simulink model "S205_Anwendungsbeispiel"  (R2018b)
settings: Solver=VariableStepAuto  StartTime=0.0  StopTime=10  MaxStep=0.001  RelTol=1e-3
values from neighbouring files (symbols this model uses):
  a = 0.031    [Parameter_S205.m]
  c = 1160    [Parameter_S205.m]
  d = 0.6    [Parameter_S205.m]
  delta_ksi = (20-(-20))/(2*r-1)    (= 1.37931034483)    [Parameter_S205.m]
  eta_c = 5*10^4    (= 50000)    [Parameter_S205.m]
  eta_d = 1.25    [Parameter_S205.m]
  eta_J1 = 0.15    [Parameter_S205.m]
  eta_J2 = 4*10^(-3)    (= 0.004)    [Parameter_S205.m]
  eta_Reib1 = 0.125    [Parameter_S205.m]
  eta_Reib2 = 0.1    [Parameter_S205.m]
  eta_theta_L = 8*10^(-6)    (= 8e-06)    [Parameter_S205.m]
  h = 0.4*10^(-3)    (= 0.0004)    [Parameter_S205.m]
  J1 = 0.166    [Parameter_S205.m]
  J2 = 0.336    [Parameter_S205.m]
  ksi = linspace(-20,20,2*r)    [Parameter_S205.m]
  l1 = 3.3    [Parameter_S205.m]
  l2 = 2.6    [Parameter_S205.m]
  l4 = 98    [Parameter_S205.m]
  sigma_norm = 1.6    [Parameter_S205.m]
  theta_S1 = 2    [Parameter_S205.m]
  theta_S2 = 38    [Parameter_S205.m]
undefined symbols (not defined in the file or in its folder): DiscIntNeverNeededParam
libraries: simulink x1
settings Model: Creator=LENOVO  LastModifiedBy=LENOVO

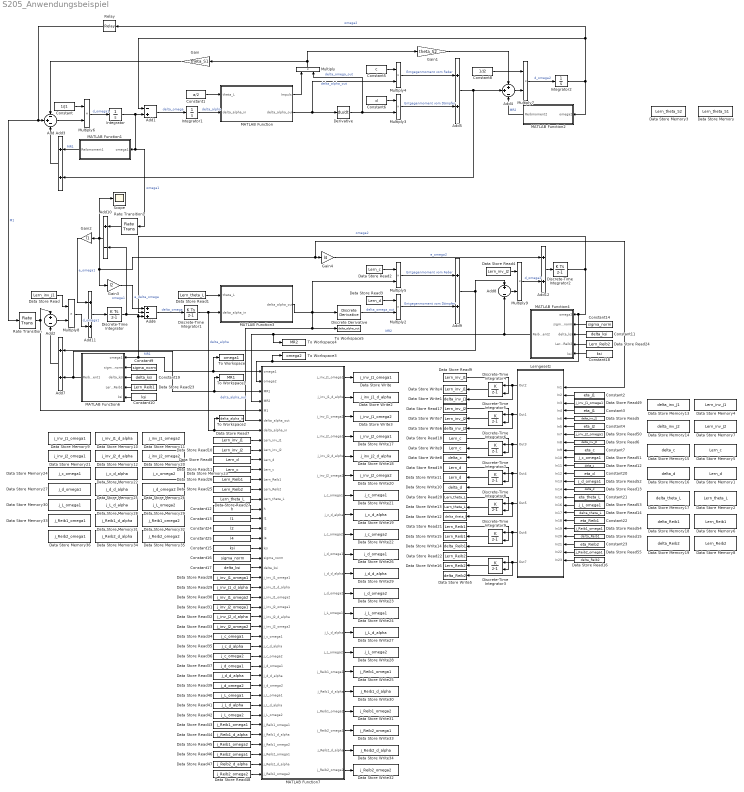
== system S205_Anwendungsbeispiel ==
  Add : Sum  Inputs=-+-
  Add1 : Sum  Inputs=-+
  Add10 : Sum  Inputs=+-
  Add{3,5,7,9,11..12} (6 alike) : Sum
  Add2 : Sum  Inputs=+-
  Add4 : Sum  Inputs=++-
  Add6 : Sum  Inputs=+-+
  Add8 : Sum  Inputs=+-
  Constant : Constant  Value=1/J1
  Constant1 : Constant  Value=a/2
  Constant10 : Constant  Value=ksi
  Constant11 : Constant  Value=delta_ksi
  Constant12 : Constant  Value=h
  Constant13 : Constant  Value=l1
  Constant14 : Constant  Value=sigma_norm
  Constant15 : Constant  Value=ksi
  Constant16 : Constant  Value=sigma_norm
  Constant17 : Constant  Value=delta_ksi
  Constant18 : Constant  Value=ksi
  Constant19 : Constant  Value=delta_ksi
  Constant2 : Constant  Value=eta_J1
  Constant20 : Constant  Value=eta_d
  Constant21 : Constant  Value=eta_theta_L
  Constant22 : Constant  Value=eta_Reib1
  Constant23 : Constant  Value=eta_Reib2
  Constant24 : Constant  Value=l2
  Constant25 : Constant  Value=l4
  Constant3 : Constant  Value=eta_J1
  Constant4 : Constant  Value=eta_J2
  Constant5 : Constant  Value=c
  Constant6 : Constant  Value=d
  Constant7 : Constant  Value=eta_c
  Constant8 : Constant  Value=1/J2
  Constant9 : Constant  Value=sigma_norm
  Data Store Memory : DataStoreMemory  DataStoreName=Lern_theta_S1  ReadBeforeWriteMsg=warning  WriteAfterWriteMsg=warning  WriteAfterReadMsg=warning  ShowAdditionalParam=off
  Data Store Memory1 : DataStoreMemory  DataStoreName=Lern_d  ReadBeforeWriteMsg=warning  WriteAfterWriteMsg=warning  WriteAfterReadMsg=warning  InitialValue=1  ShowAdditionalParam=off
  Data Store Memory10 : DataStoreMemory  DataStoreName=j_inv_J1_d_alpha  ReadBeforeWriteMsg=warning  WriteAfterWriteMsg=warning  WriteAfterReadMsg=warning  ShowAdditionalParam=off
  Data Store Memory11 : DataStoreMemory  DataStoreName=j_inv_J1_omega2  ReadBeforeWriteMsg=warning  WriteAfterWriteMsg=warning  WriteAfterReadMsg=warning  ShowAdditionalParam=off
  Data Store Memory12 : DataStoreMemory  DataStoreName=j_inv_J2_d_alpha  ReadBeforeWriteMsg=warning  WriteAfterWriteMsg=warning  WriteAfterReadMsg=warning  ShowAdditionalParam=off
  Data Store Memory13 : DataStoreMemory  DataStoreName=delta_inv_J1  ReadBeforeWriteMsg=warning  WriteAfterWriteMsg=warning  WriteAfterReadMsg=warning  ShowAdditionalParam=off
  Data Store Memory14 : DataStoreMemory  DataStoreName=delta_inv_J2  ReadBeforeWriteMsg=warning  WriteAfterWriteMsg=warning  WriteAfterReadMsg=warning  ShowAdditionalParam=off
  Data Store Memory15 : DataStoreMemory  DataStoreName=delta_c  ReadBeforeWriteMsg=warning  WriteAfterWriteMsg=warning  WriteAfterReadMsg=warning  ShowAdditionalParam=off
  Data Store Memory16 : DataStoreMemory  DataStoreName=delta_d  ReadBeforeWriteMsg=warning  WriteAfterWriteMsg=warning  WriteAfterReadMsg=warning  ShowAdditionalParam=off
  Data Store Memory17 : DataStoreMemory  DataStoreName=delta_theta_L  ReadBeforeWriteMsg=warning  WriteAfterWriteMsg=warning  WriteAfterReadMsg=warning  ShowAdditionalParam=off
  Data Store Memory18 : DataStoreMemory  DataStoreName=delta_Reib1  ReadBeforeWriteMsg=warning  WriteAfterWriteMsg=warning  WriteAfterReadMsg=warning  InitialValue=zeros(1,30)  ShowAdditionalParam=off
  Data Store Memory19 : DataStoreMemory  DataStoreName=delta_Reib2  ReadBeforeWriteMsg=warning  WriteAfterWriteMsg=warning  WriteAfterReadMsg=warning  InitialValue=zeros(1,30)  ShowAdditionalParam=off
  Data Store Memory2 : DataStoreMemory  DataStoreName=Lern_theta_L  ReadBeforeWriteMsg=warning  WriteAfterWriteMsg=warning  WriteAfterReadMsg=warning  ShowAdditionalParam=off
  Data Store Memory20 : DataStoreMemory  DataStoreName=j_inv_J2_omega2  ReadBeforeWriteMsg=warning  WriteAfterWriteMsg=warning  WriteAfterReadMsg=warning  ShowAdditionalParam=off
  Data Store Memory21 : DataStoreMemory  DataStoreName=j_inv_J2_omega1  ReadBeforeWriteMsg=warning  WriteAfterWriteMsg=warning  WriteAfterReadMsg=warning  ShowAdditionalParam=off
  Data Store Memory22 : DataStoreMemory  DataStoreName=j_c_d_alpha  ReadBeforeWriteMsg=warning  WriteAfterWriteMsg=warning  WriteAfterReadMsg=warning  ShowAdditionalParam=off
  Data Store Memory23 : DataStoreMemory  DataStoreName=j_c_omega2  ReadBeforeWriteMsg=warning  WriteAfterWriteMsg=warning  WriteAfterReadMsg=warning  ShowAdditionalParam=off
  Data Store Memory24 : DataStoreMemory  DataStoreName=j_c_omega1  ReadBeforeWriteMsg=warning  WriteAfterWriteMsg=warning  WriteAfterReadMsg=warning  ShowAdditionalParam=off
  Data Store Memory25 : DataStoreMemory  DataStoreName=j_d_d_alpha  ReadBeforeWriteMsg=warning  WriteAfterWriteMsg=warning  WriteAfterReadMsg=warning  ShowAdditionalParam=off
  Data Store Memory26 : DataStoreMemory  DataStoreName=j_d_omega2  ReadBeforeWriteMsg=warning  WriteAfterWriteMsg=warning  WriteAfterReadMsg=warning  ShowAdditionalParam=off
  Data Store Memory27 : DataStoreMemory  DataStoreName=j_d_omega1  ReadBeforeWriteMsg=warning  WriteAfterWriteMsg=warning  WriteAfterReadMsg=warning  ShowAdditionalParam=off
  Data Store Memory28 : DataStoreMemory  DataStoreName=j_L_d_alpha  ReadBeforeWriteMsg=warning  WriteAfterWriteMsg=warning  WriteAfterReadMsg=warning  ShowAdditionalParam=off
  Data Store Memory29 : DataStoreMemory  DataStoreName=j_L_omega2  ReadBeforeWriteMsg=warning  WriteAfterWriteMsg=warning  WriteAfterReadMsg=warning  ShowAdditionalParam=off
  Data Store Memory3 : DataStoreMemory  DataStoreName=Lern_theta_S2  ReadBeforeWriteMsg=warning  WriteAfterWriteMsg=warning  WriteAfterReadMsg=warning  ShowAdditionalParam=off
  Data Store Memory30 : DataStoreMemory  DataStoreName=j_L_omega1  ReadBeforeWriteMsg=warning  WriteAfterWriteMsg=warning  WriteAfterReadMsg=warning  ShowAdditionalParam=off
  Data Store Memory31 : DataStoreMemory  DataStoreName=j_Reib1_d_alpha  ReadBeforeWriteMsg=warning  WriteAfterWriteMsg=warning  WriteAfterReadMsg=warning  InitialValue=zeros(1,30)  ShowAdditionalParam=off
  Data Store Memory32 : DataStoreMemory  DataStoreName=j_Reib1_omega2  ReadBeforeWriteMsg=warning  WriteAfterWriteMsg=warning  WriteAfterReadMsg=warning  InitialValue=zeros(1,30)  ShowAdditionalParam=off
  Data Store Memory33 : DataStoreMemory  DataStoreName=j_Reib1_omega1  ReadBeforeWriteMsg=warning  WriteAfterWriteMsg=warning  WriteAfterReadMsg=warning  InitialValue=zeros(1,30)  ShowAdditionalParam=off
  Data Store Memory34 : DataStoreMemory  DataStoreName=j_Reib2_d_alpha  ReadBeforeWriteMsg=warning  WriteAfterWriteMsg=warning  WriteAfterReadMsg=warning  InitialValue=zeros(1,30)  ShowAdditionalParam=off
  Data Store Memory35 : DataStoreMemory  DataStoreName=j_Reib2_omega2  ReadBeforeWriteMsg=warning  WriteAfterWriteMsg=warning  WriteAfterReadMsg=warning  InitialValue=zeros(1,30)  ShowAdditionalParam=off
  Data Store Memory36 : DataStoreMemory  DataStoreName=j_Reib2_omega1  ReadBeforeWriteMsg=warning  WriteAfterWriteMsg=warning  WriteAfterReadMsg=warning  InitialValue=zeros(1,30)  ShowAdditionalParam=off
  Data Store Memory4 : DataStoreMemory  DataStoreName=Lern_inv_J1  ReadBeforeWriteMsg=warning  WriteAfterWriteMsg=warning  WriteAfterReadMsg=warning  InitialValue=0.2  ShowAdditionalParam=off
  Data Store Memory5 : DataStoreMemory  DataStoreName=Lern_c  ReadBeforeWriteMsg=warning  WriteAfterWriteMsg=warning  WriteAfterReadMsg=warning  InitialValue=1350  ShowAdditionalParam=off
  Data Store Memory6 : DataStoreMemory  DataStoreName=Lern_Reib1  ReadBeforeWriteMsg=warning  WriteAfterWriteMsg=warning  WriteAfterReadMsg=warning  InitialValue=zeros(1,30)  ShowAdditionalParam=off
  Data Store Memory7 : DataStoreMemory  DataStoreName=Lern_inv_J2  ReadBeforeWriteMsg=warning  WriteAfterWriteMsg=warning  WriteAfterReadMsg=warning  InitialValue=0.45  ShowAdditionalParam=off
  Data Store Memory8 : DataStoreMemory  DataStoreName=Lern_Reib2  ReadBeforeWriteMsg=warning  WriteAfterWriteMsg=warning  WriteAfterReadMsg=warning  InitialValue=zeros(1,30)  ShowAdditionalParam=off
  Data Store Memory9 : DataStoreMemory  DataStoreName=j_inv_J1_omega1  ReadBeforeWriteMsg=warning  WriteAfterWriteMsg=warning  WriteAfterReadMsg=warning  ShowAdditionalParam=off
  Data Store Read : DataStoreRead  DataStoreName=Lern_inv_J1
  Data Store Read1 : DataStoreRead  DataStoreName=Lern_theta_L
  Data Store Read10 : DataStoreRead  DataStoreName=Lern_inv_J2
  Data Store Read11 : DataStoreRead  DataStoreName=Lern_c
  Data Store Read12 : DataStoreRead  DataStoreName=delta_c
  Data Store Read13 : DataStoreRead  DataStoreName=delta_d
  Data Store Read14 : DataStoreRead  DataStoreName=delta_theta_L
  Data Store Read15 : DataStoreRead  DataStoreName=delta_Reib1
  Data Store Read16 : DataStoreRead  DataStoreName=delta_Reib2
  Data Store Read17 : DataStoreRead  DataStoreName=Lern_inv_J2
  Data Store Read18 : DataStoreRead  DataStoreName=Lern_c
  Data Store Read19 : DataStoreRead  DataStoreName=Lern_d
  Data Store Read2 : DataStoreRead  DataStoreName=Lern_c
  Data Store Read20 : DataStoreRead  DataStoreName=Lern_theta_L
  Data Store Read21 : DataStoreRead  DataStoreName=Lern_Reib1
  Data Store Read22 : DataStoreRead  DataStoreName=Lern_Reib2
  Data Store Read23 : DataStoreRead  DataStoreName=Lern_Reib1
  Data Store Read24 : DataStoreRead  DataStoreName=Lern_Reib2
  Data Store Read25 : DataStoreRead  DataStoreName=Lern_Reib2
  Data Store Read26 : DataStoreRead  DataStoreName=Lern_Reib1
  Data Store Read27 : DataStoreRead  DataStoreName=Lern_theta_L
  Data Store Read28 : DataStoreRead  DataStoreName=j_inv_J1_omega1
  Data Store Read29 : DataStoreRead  DataStoreName=j_inv_J1_d_alpha
  Data Store Read3 : DataStoreRead  DataStoreName=Lern_d
  Data Store Read30 : DataStoreRead  DataStoreName=j_inv_J1_omega2
  Data Store Read31 : DataStoreRead  DataStoreName=j_inv_J2_omega1
  Data Store Read32 : DataStoreRead  DataStoreName=j_inv_J2_d_alpha
  Data Store Read33 : DataStoreRead  DataStoreName=j_inv_J2_omega2
  Data Store Read34 : DataStoreRead  DataStoreName=j_c_omega1
  Data Store Read35 : DataStoreRead  DataStoreName=j_c_d_alpha
  Data Store Read36 : DataStoreRead  DataStoreName=j_c_omega2
  Data Store Read37 : DataStoreRead  DataStoreName=j_d_omega1
  Data Store Read38 : DataStoreRead  DataStoreName=j_d_d_alpha
  Data Store Read39 : DataStoreRead  DataStoreName=j_d_omega2
  Data Store Read4 : DataStoreRead  DataStoreName=Lern_inv_J2
  Data Store Read40 : DataStoreRead  DataStoreName=j_L_omega1
  Data Store Read41 : DataStoreRead  DataStoreName=j_L_d_alpha
  Data Store Read42 : DataStoreRead  DataStoreName=j_L_omega2
  Data Store Read43 : DataStoreRead  DataStoreName=j_Reib1_omega1
  Data Store Read44 : DataStoreRead  DataStoreName=j_Reib1_d_alpha
  Data Store Read45 : DataStoreRead  DataStoreName=j_Reib1_omega2
  Data Store Read46 : DataStoreRead  DataStoreName=j_Reib2_omega1
  Data Store Read47 : DataStoreRead  DataStoreName=j_Reib2_d_alpha
  Data Store Read48 : DataStoreRead  DataStoreName=j_Reib2_omega2
  Data Store Read49 : DataStoreRead  DataStoreName=j_inv_J1_omega1
  Data Store Read5 : DataStoreRead  DataStoreName=delta_inv_J1
  Data Store Read50 : DataStoreRead  DataStoreName=j_inv_J2_omega1
  Data Store Read51 : DataStoreRead  DataStoreName=j_c_omega1
  Data Store Read52 : DataStoreRead  DataStoreName=j_d_omega1
  Data Store Read53 : DataStoreRead  DataStoreName=j_L_omega1
  Data Store Read54 : DataStoreRead  DataStoreName=j_Reib1_omega1
  Data Store Read55 : DataStoreRead  DataStoreName=j_Reib2_omega1
  Data Store Read6 : DataStoreRead  DataStoreName=delta_inv_J2
  Data Store Read7 : DataStoreRead  DataStoreName=Lern_inv_J1
  Data Store Read8 : DataStoreRead  DataStoreName=Lern_d
  Data Store Read9 : DataStoreRead  DataStoreName=Lern_inv_J1
  Data Store Write : DataStoreWrite  DataStoreName=j_inv_J1_omega1
  Data Store Write1 : DataStoreWrite  DataStoreName=delta_inv_J1
  Data Store Write10 : DataStoreWrite  DataStoreName=delta_d
  Data Store Write11 : DataStoreWrite  DataStoreName=Lern_d
  Data Store Write12 : DataStoreWrite  DataStoreName=delta_theta_L
  Data Store Write13 : DataStoreWrite  DataStoreName=Lern_theta_L
  Data Store Write14 : DataStoreWrite  DataStoreName=delta_Reib1
  Data Store Write15 : DataStoreWrite  DataStoreName=Lern_Reib1
  Data Store Write16 : DataStoreWrite  DataStoreName=Lern_Reib2
  Data Store Write17 : DataStoreWrite  DataStoreName=j_inv_J2_omega1
  Data Store Write18 : DataStoreWrite  DataStoreName=j_inv_J2_d_alpha
  Data Store Write19 : DataStoreWrite  DataStoreName=j_c_d_alpha
  Data Store Write2 : DataStoreWrite  DataStoreName=j_inv_J1_d_alpha
  Data Store Write20 : DataStoreWrite  DataStoreName=j_inv_J2_omega2
  Data Store Write21 : DataStoreWrite  DataStoreName=j_c_omega1
  Data Store Write22 : DataStoreWrite  DataStoreName=j_c_omega2
  Data Store Write23 : DataStoreWrite  DataStoreName=j_d_omega2
  Data Store Write24 : DataStoreWrite  DataStoreName=j_L_omega1
  Data Store Write25 : DataStoreWrite  DataStoreName=j_Reib1_omega1
  Data Store Write26 : DataStoreWrite  DataStoreName=j_d_omega1
  Data Store Write27 : DataStoreWrite  DataStoreName=j_L_d_alpha
  Data Store Write28 : DataStoreWrite  DataStoreName=j_L_omega2
  Data Store Write29 : DataStoreWrite  DataStoreName=j_d_d_alpha
  Data Store Write3 : DataStoreWrite  DataStoreName=j_inv_J1_omega2
  Data Store Write30 : DataStoreWrite  DataStoreName=j_Reib1_d_alpha
  Data Store Write31 : DataStoreWrite  DataStoreName=j_Reib1_omega2
  Data Store Write32 : DataStoreWrite  DataStoreName=j_Reib2_omega2
  Data Store Write33 : DataStoreWrite  DataStoreName=j_Reib2_omega1
  Data Store Write34 : DataStoreWrite  DataStoreName=j_Reib2_d_alpha
  Data Store Write4 : DataStoreWrite  DataStoreName=Lern_inv_J1
  Data Store Write5 : DataStoreWrite  DataStoreName=delta_Reib2
  Data Store Write6 : DataStoreWrite  DataStoreName=delta_inv_J2
  Data Store Write7 : DataStoreWrite  DataStoreName=Lern_inv_J2
  Data Store Write8 : DataStoreWrite  DataStoreName=delta_c
  Data Store Write9 : DataStoreWrite  DataStoreName=Lern_c
  Derivative : Derivative
  Discrete Derivative : simulink/Discrete/Discrete Derivative  gainval=1.0  ICPrevScaledInput=0.0  OutMin=[]  OutMax=[]  OutDataType=fixdt(1, 16)  OutScaling=2^-10  DoSatur=off
  Discrete-Time Integrator : DiscreteIntegrator  SampleTime=-1  ICPrevOutput=DiscIntNeverNeededParam  ICPrevScaledInput=DiscIntNeverNeededParam
  Discrete-Time Integrator1 : DiscreteIntegrator  SampleTime=-1  ICPrevOutput=DiscIntNeverNeededParam  ICPrevScaledInput=DiscIntNeverNeededParam
  Discrete-Time Integrator2 : DiscreteIntegrator  InitialCondition=-20  SampleTime=0.004  ICPrevOutput=DiscIntNeverNeededParam  ICPrevScaledInput=DiscIntNeverNeededParam
  Discrete-Time Integrator{3..9} (7 alike) : DiscreteIntegrator  IntegratorMethod=Accumulation: Forward Euler  InitialConditionSource=external  SampleTime=-1  ICPrevOutput=DiscIntNeverNeededParam  ICPrevScaledInput=DiscIntNeverNeededParam
  Gain : Gain  Gain=theta_S1
  Gain1 : Gain  Gain=theta_S2
  Gain2 : Gain  Gain=l1
  Gain3 : Gain  Gain=l2
  Gain4 : Gain  Gain=l4
  Integrator : Integrator
  Integrator1 : Integrator
  Integrator2 : Integrator  InitialCondition=-20
  Lerngesetz : Subsystem
  MATLAB Function : MATLAB Function  TreatAsAtomicUnit=on
  MATLAB Function1 : MATLAB Function  TreatAsAtomicUnit=on
  MATLAB Function2 : MATLAB Function  TreatAsAtomicUnit=on
  MATLAB Function3 : MATLAB Function  TreatAsAtomicUnit=on
  MATLAB Function4 : MATLAB Function  TreatAsAtomicUnit=on
  MATLAB Function6 : MATLAB Function  TreatAsAtomicUnit=on
  MATLAB Function7 : MATLAB Function  TreatAsAtomicUnit=on
  Multiply{,2..9} (9 alike) : Product
  Rate Transition : RateTransition  OutPortSampleTime=0.004
  Rate Transition1 : RateTransition  OutPortSampleTime=0.004
  Relay : Relay  OnSwitchValue=20  OffSwitchValue=-20  OnOutputValue=-10  OffOutputValue=10
  Scope : Scope
  To Workspace : ToWorkspace  VariableName=omega1  SaveFormat=Timeseries  SampleTime=-1
  To Workspace1 : ToWorkspace  VariableName=MR1  SaveFormat=Timeseries  SampleTime=-1
  To Workspace2 : ToWorkspace  VariableName=delta_alpha_in  SaveFormat=Timeseries  SampleTime=-1
  To Workspace3 : ToWorkspace  VariableName=omega2  SaveFormat=Timeseries  SampleTime=-1
  To Workspace4 : ToWorkspace  VariableName=MR2  SaveFormat=Timeseries  SampleTime=-1
  To Workspace5 : ToWorkspace  VariableName=delta_alpha_out  SaveFormat=Timeseries  SampleTime=-1
  wires:
  Add1/1 -> Integrator1/1  "delta_omega"
  Integrator1/1 -> MATLAB Function/2(delta_alpha_in)  "delta_alpha"
  MATLAB Function/2(delta_alpha_out) -> Derivative/1, Multiply4/2  "delta_alpha_out"
  Derivative/1 -> Multiply/2, Multiply3/2  "delta_omega_out"
  Integrator/1 -> Rate Transition1/1, MATLAB Function1/1(omega1), Add1/2  "omega1"
  MATLAB Function1/1(Reibmoment1) -> Add3/1  "MR1"
  Constant6/1 -> Multiply3/1
  Constant5/1 -> Multiply4/1
  Multiply4/1 -> Add5/1  "Entgegenmoment vom Feder"
  Multiply3/1 -> Add5/2  "Entgegenmoment vom Dämpfer"
  Multiply6/1 -> Integrator/1  "d_omega1"
  Add/1 -> Multiply6/2
  Constant/1 -> Multiply6/1
  Add4/1 -> Multiply7/2
  Constant8/1 -> Multiply7/1
  Multiply7/1 -> Integrator2/1  "d_omega2"
  Integrator2/1 -> Add1/1, Relay/1, MATLAB Function2/1(omega2)  "omega2"
  Constant1/1 -> MATLAB Function/1(theta_L)
  Add5/1 -> Add4/2, Add3/2
  Add3/1 -> Add/3
  Relay/1 -> Rate Transition/1, Add/2  "M1"
  MATLAB Function/1(Impuls) -> Multiply/1
  Multiply/1 -> Gain1/1, Gain/1
  Gain/1 -> Add/1
  MATLAB Function2/1(Reibmoment2) -> Add4/3  "MR2"
  Gain1/1 -> Add4/1
  MATLAB Function4/1(Reibmoment2) -> To Workspace4/1, MATLAB Function7/4(MR2), Add8/2  "MR2"
  Add7/1 -> Add2/2
  Add9/1 -> Add7/1, Add8/1
  Data Store Read1/1 -> MATLAB Function3/1(theta_L)
  Discrete-Time Integrator2/1 -> To Workspace3/1, MATLAB Function7/2(omega2), MATLAB Function4/1(omega2), Add6/2  "omega2"
  Multiply9/1 -> Add12/2  "d_omega2"
  Data Store Read4/1 -> Multiply9/1
  Add8/1 -> Multiply9/2
  Data Store Read/1 -> Multiply8/1
  Add2/1 -> Multiply8/2
  Multiply2/1 -> Add9/2  "Entgegenmoment vom Dämpfer"
  Multiply5/1 -> Add9/1  "Entgegenmoment vom Feder"
  Data Store Read2/1 -> Multiply5/1
  Data Store Read3/1 -> Multiply2/1
  Discrete-Time Integrator/1 -> To Workspace/1, MATLAB Function7/1(omega1), MATLAB Function6/1(omega1), Add6/3, Add10/2  "omega1"
  Discrete Derivative/1 -> Multiply2/2  "delta_omega_out"
  MATLAB Function3/1(delta_alpha_out) -> To Workspace5/1, MATLAB Function7/6(delta_alpha_out), Multiply5/2, Discrete Derivative/1  "delta_alpha_out"
  Discrete-Time Integrator1/1 -> To Workspace2/1, MATLAB Function7/7(delta_alpha_in), MATLAB Function3/2(delta_alpha_in)  "delta_alpha"
  Add6/1 -> Discrete-Time Integrator1/1  "delta_omega"
  Rate Transition/1 -> MATLAB Function7/5(M1), Add2/1
  Rate Transition1/1 -> Add10/1
  Add11/1 -> Discrete-Time Integrator/1
  Multiply8/1 -> Add11/2  "d_omega1"
  Add10/1 -> Lerngesetz/1(In1), Gain4/1, Gain3/1, Scope/1, Gain2/1
  Gain2/1 -> Add11/1  "e_omega1"
  Constant17/1 -> MATLAB Function7/21(delta_ksi)
  Constant12/1 -> MATLAB Function7/15(h)
  Constant10/1 -> MATLAB Function6/5(ksi)
  Constant16/1 -> MATLAB Function7/20(sigma_norm)
  Data Store Read9/1 -> Discrete-Time Integrator4/2
  Constant15/1 -> MATLAB Function7/19(ksi)
  Discrete-Time Integrator4/1 -> Data Store Write4/1
  Constant9/1 -> MATLAB Function6/2(sigma_norm)
  Constant19/1 -> MATLAB Function6/3(delta_ksi)
  MATLAB Function6/1(Reibmoment1) -> To Workspace1/1, MATLAB Function7/3(MR1), Add7/2  "MR1"
  Gain3/1 -> Add6/1  "e_delta_omega"
  Add12/1 -> Discrete-Time Integrator2/1
  Gain4/1 -> Add12/1  "e_omega2"
  Constant11/1 -> MATLAB Function4/3(delta_ksi)
  Constant14/1 -> MATLAB Function4/2(sigma_norm)
  Constant18/1 -> MATLAB Function4/5(ksi)
  Constant2/1 -> Lerngesetz/2(In2)
  Constant3/1 -> Lerngesetz/4(In4)
  Constant4/1 -> Lerngesetz/6(In5)
  Constant7/1 -> Lerngesetz/9(In9)
  Constant20/1 -> Lerngesetz/12(In12)
  Constant21/1 -> Lerngesetz/15(In15)
  Data Store Read5/1 -> Lerngesetz/5(In6)
  Data Store Read6/1 -> Lerngesetz/8(In8)
  Data Store Read12/1 -> Lerngesetz/11(In11)
  Data Store Read13/1 -> Lerngesetz/14(In14)
  Constant22/1 -> Lerngesetz/18(In18)
  Constant23/1 -> Lerngesetz/21(In21)
  Data Store Read14/1 -> Lerngesetz/17(In17)
  Data Store Read15/1 -> Lerngesetz/20(In20)
  Data Store Read16/1 -> Lerngesetz/23(In23)
  Lerngesetz/1(Out2) -> Discrete-Time Integrator4/1, Data Store Write1/1
  Lerngesetz/2(Out1) -> Discrete-Time Integrator5/1, Data Store Write6/1
  Discrete-Time Integrator5/1 -> Data Store Write7/1
  Data Store Read17/1 -> Discrete-Time Integrator5/2
  Data Store Read18/1 -> Discrete-Time Integrator6/2
  Discrete-Time Integrator6/1 -> Data Store Write9/1
  Lerngesetz/3(Out3) -> Data Store Write8/1, Discrete-Time Integrator6/1
  Lerngesetz/4(Out4) -> Discrete-Time Integrator7/1, Data Store Write10/1
  Discrete-Time Integrator7/1 -> Data Store Write11/1
  Data Store Read19/1 -> Discrete-Time Integrator7/2
  Data Store Read20/1 -> Discrete-Time Integrator8/2
  Discrete-Time Integrator8/1 -> Data Store Write13/1
  Lerngesetz/5(Out5) -> Data Store Write12/1, Discrete-Time Integrator8/1
  Lerngesetz/6(Out6) -> Discrete-Time Integrator9/1, Data Store Write14/1
  Discrete-Time Integrator9/1 -> Data Store Write15/1
  Data Store Read21/1 -> Discrete-Time Integrator9/2
  Data Store Read22/1 -> Discrete-Time Integrator3/2
  Discrete-Time Integrator3/1 -> Data Store Write16/1
  Lerngesetz/7(Out7) -> Data Store Write5/1, Discrete-Time Integrator3/1
  Data Store Read23/1 -> MATLAB Function6/4(Lern_Reib1)
  Data Store Read24/1 -> MATLAB Function4/4(Lern_Reib2)
  MATLAB Function7/1(j_inv_J1_omega1) -> Data Store Write/1
  MATLAB Function7/2(j_inv_J1_d_alpha) -> Data Store Write2/1
  MATLAB Function7/3(j_inv_J1_omega2) -> Data Store Write3/1
  MATLAB Function7/4(j_inv_J2_omega1) -> Data Store Write17/1
  MATLAB Function7/5(j_inv_J2_d_alpha) -> Data Store Write18/1
  MATLAB Function7/6(j_inv_J2_omega2) -> Data Store Write20/1
  MATLAB Function7/7(j_c_omega1) -> Data Store Write21/1
  MATLAB Function7/8(j_c_d_alpha) -> Data Store Write19/1
  MATLAB Function7/16(j_Reib1_omega1) -> Data Store Write25/1
  MATLAB Function7/15(j_L_omega2) -> Data Store Write28/1
  MATLAB Function7/14(j_L_d_alpha) -> Data Store Write27/1
  MATLAB Function7/13(j_L_omega1) -> Data Store Write24/1
  MATLAB Function7/12(j_d_omega2) -> Data Store Write23/1
  MATLAB Function7/11(j_d_d_alpha) -> Data Store Write29/1
  MATLAB Function7/10(j_d_omega1) -> Data Store Write26/1
  MATLAB Function7/9(j_c_omega2) -> Data Store Write22/1
  MATLAB Function7/17(j_Reib1_d_alpha) -> Data Store Write30/1
  MATLAB Function7/18(j_Reib1_omega2) -> Data Store Write31/1
  MATLAB Function7/19(j_Reib2_omega1) -> Data Store Write33/1
  MATLAB Function7/20(j_Reib2_d_alpha) -> Data Store Write34/1
  MATLAB Function7/21(j_Reib2_omega2) -> Data Store Write32/1
  Constant13/1 -> MATLAB Function7/16(l1)
  Constant24/1 -> MATLAB Function7/17(l2)
  Constant25/1 -> MATLAB Function7/18(l4)
  Data Store Read11/1 -> MATLAB Function7/11(Lern_c)
  Data Store Read8/1 -> MATLAB Function7/10(Lern_d)
  Data Store Read7/1 -> MATLAB Function7/8(Lern_inv_J1)
  Data Store Read10/1 -> MATLAB Function7/9(Lern_inv_J2)
  Data Store Read26/1 -> MATLAB Function7/12(Lern_Reib1)
  Data Store Read25/1 -> MATLAB Function7/13(Lern_Reib2)
  Data Store Read27/1 -> MATLAB Function7/14(Lern_theta_L)
  Data Store Read28/1 -> MATLAB Function7/22("j_inv_J1_omega1 ")
  Data Store Read29/1 -> MATLAB Function7/23("j_inv_J1_d_alpha ")
  Data Store Read30/1 -> MATLAB Function7/24("j_inv_J1_omega2 ")
  Data Store Read33/1 -> MATLAB Function7/27("j_inv_J2_omega2 ")
  Data Store Read32/1 -> MATLAB Function7/26("j_inv_J2_d_alpha ")
  Data Store Read31/1 -> MATLAB Function7/25("j_inv_J2_omega1 ")
  Data Store Read36/1 -> MATLAB Function7/30("j_c_omega2 ")
  Data Store Read35/1 -> MATLAB Function7/29("j_c_d_alpha ")
  Data Store Read34/1 -> MATLAB Function7/28("j_c_omega1 ")
  Data Store Read39/1 -> MATLAB Function7/33("j_d_omega2 ")
  Data Store Read38/1 -> MATLAB Function7/32("j_d_d_alpha ")
  Data Store Read37/1 -> MATLAB Function7/31("j_d_omega1 ")
  Data Store Read42/1 -> MATLAB Function7/36("j_L_omega2 ")
  Data Store Read41/1 -> MATLAB Function7/35("j_L_d_alpha ")
  Data Store Read40/1 -> MATLAB Function7/34("j_L_omega1 ")
  Data Store Read45/1 -> MATLAB Function7/39("j_Reib1_omega2 ")
  Data Store Read44/1 -> MATLAB Function7/38("j_Reib1_d_alpha ")
  Data Store Read43/1 -> MATLAB Function7/37("j_Reib1_omega1 ")
  Data Store Read48/1 -> MATLAB Function7/42("j_Reib2_omega2 ")
  Data Store Read47/1 -> MATLAB Function7/41("j_Reib2_d_alpha ")
  Data Store Read46/1 -> MATLAB Function7/40("j_Reib2_omega1 ")
  Data Store Read49/1 -> Lerngesetz/3(In3)
  Data Store Read50/1 -> Lerngesetz/7(In7)
  Data Store Read51/1 -> Lerngesetz/10(In10)
  Data Store Read52/1 -> Lerngesetz/13(In13)
  Data Store Read53/1 -> Lerngesetz/16(In16)
  Data Store Read54/1 -> Lerngesetz/19(In19)
  Data Store Read55/1 -> Lerngesetz/22(In22)

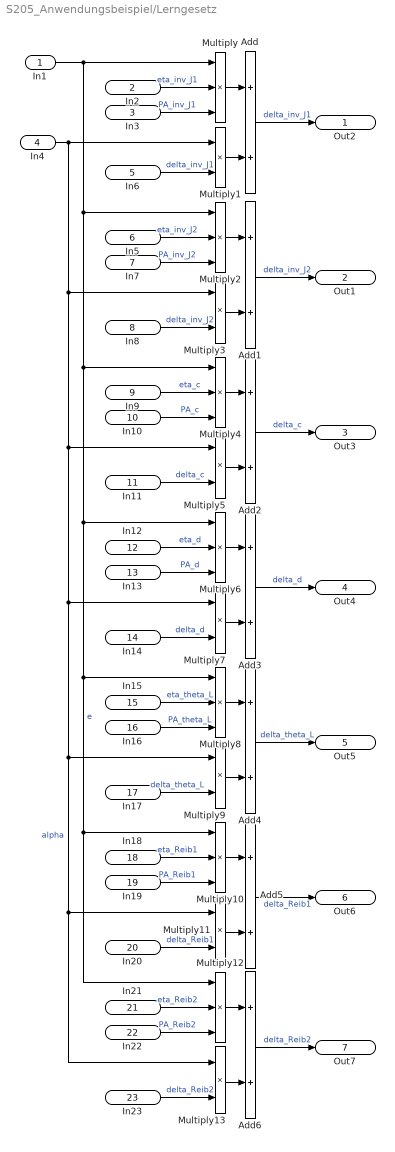
== system S205_Anwendungsbeispiel/Lerngesetz ==
  In1 : Inport
  In2 : Inport  Port=2
  In3 : Inport  Port=3
  In4 : Inport  Port=4
  In6 : Inport  Port=5
  In5 : Inport  Port=6
  In7 : Inport  Port=7
  In8 : Inport  Port=8
  In9 : Inport  Port=9
  In10 : Inport  Port=10
  In11 : Inport  Port=11
  In12 : Inport  Port=12
  In13 : Inport  Port=13
  In14 : Inport  Port=14
  In15 : Inport  Port=15
  In16 : Inport  Port=16
  In17 : Inport  Port=17
  In18 : Inport  Port=18
  In19 : Inport  Port=19
  In20 : Inport  Port=20
  In21 : Inport  Port=21
  In22 : Inport  Port=22
  In23 : Inport  Port=23
  Add{,1..6} (7 alike) : Sum  Inputs=2
  Multiply{,2,4,6,8,10,12} (7 alike) : Product  Inputs=3
  Multiply{1,3,5,7,9,11,13} (7 alike) : Product
  Out2 : Outport
  Out1 : Outport  Port=2
  Out3 : Outport  Port=3
  Out4 : Outport  Port=4
  Out5 : Outport  Port=5
  Out6 : Outport  Port=6
  Out7 : Outport  Port=7
  wires:
  In3/1 -> Multiply/3  "PA_inv_J1"
  In2/1 -> Multiply/2  "eta_inv_J1"
  In6/1 -> Multiply1/2  "delta_inv_J1"
  Multiply1/1 -> Add/2
  Multiply/1 -> Add/1
  Add/1 -> Out2/1  "delta_inv_J1"
  Add1/1 -> Out1/1  "delta_inv_J2"
  Multiply2/1 -> Add1/1
  Multiply3/1 -> Add1/2
  In8/1 -> Multiply3/2  "delta_inv_J2"
  In5/1 -> Multiply2/2  "eta_inv_J2"
  In7/1 -> Multiply2/3  "PA_inv_J2"
  In10/1 -> Multiply4/3  "PA_c"
  In9/1 -> Multiply4/2  "eta_c"
  In11/1 -> Multiply5/2  "delta_c"
  Multiply5/1 -> Add2/2
  Multiply4/1 -> Add2/1
  Add2/1 -> Out3/1  "delta_c"
  Add3/1 -> Out4/1  "delta_d"
  Multiply6/1 -> Add3/1
  Multiply7/1 -> Add3/2
  In14/1 -> Multiply7/2  "delta_d"
  In12/1 -> Multiply6/2  "eta_d"
  In13/1 -> Multiply6/3  "PA_d"
  In16/1 -> Multiply8/3  "PA_theta_L"
  In15/1 -> Multiply8/2  "eta_theta_L"
  In17/1 -> Multiply9/2  "delta_theta_L"
  Multiply9/1 -> Add4/2
  Multiply8/1 -> Add4/1
  Add4/1 -> Out5/1  "delta_theta_L"
  Add5/1 -> Out6/1  "delta_Reib1"
  Multiply10/1 -> Add5/1
  Multiply11/1 -> Add5/2
  In20/1 -> Multiply11/2  "delta_Reib1"
  In18/1 -> Multiply10/2  "eta_Reib1"
  In19/1 -> Multiply10/3  "PA_Reib1"
  In4/1 -> Multiply13/1, Multiply11/1, Multiply9/1, Multiply7/1, Multiply5/1, Multiply3/1, Multiply1/1  "alpha"
  In22/1 -> Multiply12/3  "PA_Reib2"
  In21/1 -> Multiply12/2  "eta_Reib2"
  In1/1 -> Multiply/1, Multiply12/1, Multiply10/1, Multiply8/1, Multiply6/1, Multiply4/1, Multiply2/1  "e"
  In23/1 -> Multiply13/2  "delta_Reib2"
  Multiply13/1 -> Add6/2
  Multiply12/1 -> Add6/1
  Add6/1 -> Out7/1  "delta_Reib2"

== matlab function S205_Anwendungsbeispiel/MATLAB Function1 ==
  data: omega1 input; Reibmoment1 output
function Reibmoment1=Reib1(omega1)

if omega1>0
    Reibmoment1=0.29*atan(0.3*omega1)+0.4;
elseif omega1<0
    Reibmoment1=0.35*atan(0.3*omega1)-0.15;
else
    Reibmoment1=0;
end

end

== matlab function S205_Anwendungsbeispiel/MATLAB Function ==
  data: Impuls output; theta_L input; delta_alpha_out output; delta_alpha_in input
function [Impuls,delta_alpha_out]=Losemodellierung(theta_L,delta_alpha_in)

if delta_alpha_in>theta_L
    delta_alpha_out=delta_alpha_in-theta_L;
elseif delta_alpha_in<-theta_L
    delta_alpha_out=delta_alpha_in+theta_L;
else
    delta_alpha_out=0;
end

if delta_alpha_in==theta_L || delta_alpha_in==-theta_L
    Impuls=1;
else
    Impuls=0;
end

end

== matlab function S205_Anwendungsbeispiel/MATLAB Function2 ==
  data: omega2 input; Reibmoment2 output
function Reibmoment2=Reib2(omega2)

if omega2>0
    Reibmoment2=0.29*atan(0.2*omega2)+0.3;
elseif omega2<0
    Reibmoment2=0.35*atan(0.15*omega2)-0.2;
else
    Reibmoment2=0;
end

end

== matlab function S205_Anwendungsbeispiel/MATLAB Function3 ==
  data: theta_L input; delta_alpha_out output; delta_alpha_in input
function delta_alpha_out=Losemodellierung(theta_L,delta_alpha_in)

if delta_alpha_in>theta_L
    delta_alpha_out=delta_alpha_in-theta_L;
elseif delta_alpha_in<-theta_L
    delta_alpha_out=delta_alpha_in+theta_L;
else
    delta_alpha_out=0;
end

end

== matlab function S205_Anwendungsbeispiel/MATLAB Function4 ==
  data: omega2 input; sigma_norm input; delta_ksi input; Lern_Reib2 input; Reibmoment2 output; ksi input
function Reibmoment2=Reib2(omega2,sigma_norm,delta_ksi,Lern_Reib2,ksi)

Zaehler_AF_GRNN=@(u,ksi) exp(-(u-ksi).^2/(2*sigma_norm^2*delta_ksi^2));
Nenner_AF_GRNN=@(u,ksi) sum(Zaehler_AF_GRNN(u,ksi));
AF_GRNN=@(u,ksi) Zaehler_AF_GRNN(u,ksi)/Nenner_AF_GRNN(u,ksi); %Aktivierungsfunktionen

Reibmoment2=sum(Lern_Reib2.*AF_GRNN(omega2,ksi));

end

== matlab function S205_Anwendungsbeispiel/MATLAB Function6 ==
  data: omega1 input; sigma_norm input; delta_ksi input; Lern_Reib1 input; Reibmoment1 output; ksi input
function Reibmoment1=Reib1(omega1,sigma_norm,delta_ksi,Lern_Reib1,ksi)

Zaehler_AF_GRNN=@(u,ksi) exp(-(u-ksi).^2/(2*sigma_norm^2*delta_ksi^2));
Nenner_AF_GRNN=@(u,ksi) sum(Zaehler_AF_GRNN(u,ksi));
AF_GRNN=@(u,ksi) Zaehler_AF_GRNN(u,ksi)/Nenner_AF_GRNN(u,ksi); %Aktivierungsfunktionen

Reibmoment1=sum(Lern_Reib1.*AF_GRNN(omega1,ksi));

end

== matlab function S205_Anwendungsbeispiel/MATLAB Function7 ==
  data: omega1 input; omega2 input; MR1 input; MR2 input; M1 input; delta_alpha_out input; delta_alpha_in input; j_inv_J1_omega1 output; Lern_inv_J1 input; Lern_inv_J2 input; Lern_d input; Lern_c input; Lern_Reib1 input; Lern_Reib2 input; Lern_theta_L input; j_inv_J1_d_alpha output; h input; l1 input; l2 input; l4 input; ksi input; sigma_norm input; delta_ksi input; j_inv_J1_omega2 output; j_inv_J2_omega1 output; j_inv_J2_d_alpha output; j_inv_J2_omega2 output; j_c_omega1 output; j_c_d_alpha output; j_c_omega2 output; j_d_omega1 output; j_d_d_alpha output; j_d_omega2 output; j_L_omega1 output; j_L_d_alpha output; j_L_omega2 output; j_Reib1_omega1 output; j_Reib1_d_alpha output; j_Reib1_omega2 output; j_Reib2_omega1 output; j_Reib2_d_alpha output; j_Reib2_omega2 output; j_inv_J1_omega1 input; j_inv_J1_d_alpha input; j_inv_J1_omega2 input; j_inv_J2_omega1 input; j_inv_J2_d_alpha input; j_inv_J2_omega2 input; j_c_omega1 input; j_c_d_alpha input; j_c_omega2 input; j_d_omega1 input; j_d_d_alpha input; j_d_omega2 input; j_L_omega1 input; j_L_d_alpha input; j_L_omega2 input; j_Reib1_omega1 input; j_Reib1_d_alpha input; j_Reib1_omega2 input; j_Reib2_omega1 input; j_Reib2_d_alpha input; j_Reib2_omega2 input
function [j_inv_J1_omega1,j_inv_J1_d_alpha,j_inv_J1_omega2,j_inv_J2_omega1,j_inv_J2_d_alpha,j_inv_J2_omega2,j_c_omega1,j_c_d_alpha,j_c_omega2,j_d_omega1,j_d_d_alpha,j_d_omega2,j_L_omega1,j_L_d_alpha,j_L_omega2,j_Reib1_omega1,j_Reib1_d_alpha,j_Reib1_omega2,j_Reib2_omega1,j_Reib2_d_alpha,j_Reib2_omega2]=Partielle_Ableitung(omega1,omega2,MR1,MR2,M1,delta_alpha_out,delta_alpha_in,Lern_inv_J1,Lern_inv_J2,Lern_d,Lern_c,Lern_Reib1,Lern_Reib2,Lern_theta_L,h,l1,l2,l4,ksi,sigma_norm,delta_ksi,j_inv_J1_omega1,j_inv_J1_d_alpha,j_inv_J1_omega2,j_inv_J2_omega1,j_inv_J2_d_alpha,j_inv_J2_omega2,j_c_omega1,j_c_d_alpha,j_c_omega2,j_d_omega1,j_d_d_alpha,j_d_omega2,j_L_omega1,j_L_d_alpha,j_L_omega2,j_Reib1_omega1,j_Reib1_d_alpha,j_Reib1_omega2,j_Reib2_omega1,j_Reib2_d_alpha,j_Reib2_omega2)

% Aktivierungsfunktionen
Zaehler_AF_GRNN=@(u,ksi) exp(-(u-ksi).^2/(2*sigma_norm^2*delta_ksi^2));
Nenner_AF_GRNN=@(u,ksi) sum(Zaehler_AF_GRNN(u,ksi));
AF_GRNN=@(u,ksi) Zaehler_AF_GRNN(u,ksi)/Nenner_AF_GRNN(u,ksi);

% partielle Ableitung des Reibapproximators
Grad_Reib1=0;
for j=1:30
    Grad_Reib1=Grad_Reib1+AF_GRNN(omega1,ksi(j))*(omega1-ksi(j))/(sigma_norm^2*delta_ksi^2)*(MR1-Lern_Reib1(j));
end

Grad_Reib2=0;
for j=1:30
    Grad_Reib2=Grad_Reib2+AF_GRNN(omega2,ksi(j))*(omega2-ksi(j))/(sigma_norm^2*delta_ksi^2)*(MR2-Lern_Reib2(j));
end

% partielle Ableitung des Loseapproximators
Grad_alpha_out_inv_J1=0;
Grad_alpha_out_inv_J2=0;
Grad_alpha_out_c=0;
Grad_alpha_out_d=0;
Grad_alpha_out_Reib1=zeros(30,1);
Grad_alpha_out_Reib2=zeros(30,1);
Grad_alpha_out_L=0;

if delta_alpha_in>Lern_theta_L
    Grad_alpha_out_inv_J1=j_inv_J1_d_alpha;
    Grad_alpha_out_inv_J2=j_inv_J2_d_alpha;
    Grad_alpha_out_c=j_c_d_alpha;
    Grad_alpha_out_d=j_d_d_alpha;
    Grad_alpha_out_Reib1=j_Reib1_d_alpha;
    Grad_alpha_out_Reib2=j_Reib2_d_alpha;
    Grad_alpha_out_L=j_L_d_alpha-1;
elseif delta_alpha_in<-Lern_theta_L
    Grad_alpha_out_inv_J1=j_inv_J1_d_alpha;
    Grad_alpha_out_inv_J2=j_inv_J2_d_alpha;
    Grad_alpha_out_c=j_c_d_alpha;
    Grad_alpha_out_d=j_d_d_alpha;
    Grad_alpha_out_Reib1=j_Reib1_d_alpha;
    Grad_alpha_out_Reib2=j_Reib2_d_alpha;
    Grad_alpha_out_L=j_L_d_alpha+1;
else
    Grad_alpha_out_inv_J1=0;
    Grad_alpha_out_inv_J2=0;
    Grad_alpha_out_c=0;
    Grad_alpha_out_d=0;
    Grad_alpha_out_Reib1=zeros(30,1);
    Grad_alpha_out_Reib2=zeros(30,1);
    Grad_alpha_out_L=0;
end

% j-Parameter abhaengig von d_alpha
j_inv_J1_d_alpha=j_inv_J1_d_alpha+h*(l2+1)*j_inv_J1_omega1-h*j_inv_J1_omega2;
j_inv_J2_d_alpha=j_inv_J2_d_alpha+h*(l2+1)*j_inv_J2_omega1-h*j_inv_J2_omega2;
j_c_d_alpha=j_c_d_alpha+h*(l2+1)*j_c_omega1-h*j_c_omega2;
j_d_d_alpha=j_d_d_alpha+h*(l2+1)*j_d_omega1-h*j_d_omega2;
j_Reib1_d_alpha=j_Reib1_d_alpha+h.*(l2+1).*j_Reib1_omega1-h.*j_Reib1_omega2;
j_Reib2_d_alpha=j_Reib2_d_alpha+h.*(l2+1).*j_Reib2_omega1-h.*j_Reib2_omega2;
j_L_d_alpha=j_L_d_alpha+h*(l2+1)*j_L_omega1-h*j_L_omega2;

% j-Parameter abhaengig von omega2
j_inv_J1_omega2=j_inv_J1_omega2+h*l4*j_inv_J1_omega1-h*Lern_inv_J2*j_inv_J1_omega2*Grad_Reib2+(h*Lern_c*Lern_inv_J2+Lern_d*Lern_inv_J2)*Grad_alpha_out_inv_J1;
j_inv_J2_omega2=j_inv_J2_omega2+h*l4*j_inv_J2_omega1-h*MR2-h*Lern_inv_J2*j_inv_J2_omega2*Grad_Reib2+(h*Lern_c+Lern_d)*delta_alpha_out+(h*Lern_c*Lern_inv_J2+Lern_d*Lern_inv_J2)*Grad_alpha_out_inv_J2;
j_c_omega2=j_c_omega2+h*l4*j_c_omega1-h*Lern_inv_J2*j_c_omega2*Grad_Reib2+h*Lern_inv_J2*delta_alpha_out+(h*Lern_c*Lern_inv_J2+Lern_d*Lern_inv_J2)*Grad_alpha_out_c;
j_d_omega2=j_d_omega2+h*l4*j_d_omega1-h*Lern_inv_J2*j_d_omega2*Grad_Reib2+Lern_inv_J2*delta_alpha_out+(h*Lern_c*Lern_inv_J2+Lern_d*Lern_inv_J2)*Grad_alpha_out_d;
j_Reib1_omega2=j_Reib1_omega2+h.*l4.*j_Reib1_omega1-h.*Lern_inv_J2.*Grad_Reib2.*j_Reib1_omega2+(h.*Lern_c.*Lern_inv_J2+Lern_d.*Lern_inv_J2).*Grad_alpha_out_Reib1;
j_Reib2_omega2=j_Reib2_omega2+h.*l4.*j_Reib2_omega1-h.*Lern_inv_J2.*(AF_GRNN(omega2,ksi)+j_Reib2_omega2.*Grad_Reib2)+(h.*Lern_c.*Lern_inv_J2+Lern_d.*Lern_inv_J2).*Grad_alpha_out_Reib2;
j_L_omega2=j_L_omega2+h*l4*j_L_omega1-h*Lern_inv_J2*j_L_omega2*Grad_Reib2+(h*Lern_c*Lern_inv_J2+Lern_d*Lern_inv_J2)*Grad_alpha_out_L;

% j-Parameter abhaengig von omega1
j_inv_J1_omega1=(1+h*l1)*j_inv_J1_omega1+h*M1-h*MR1-h*Lern_inv_J1*j_inv_J1_omega1*Grad_Reib1-(h*Lern_c+Lern_d)*delta_alpha_out-(h*Lern_inv_J1*Lern_c+Lern_inv_J1*Lern_d)*Grad_alpha_out_inv_J1;
j_inv_J2_omega1=(1+h*l1)*j_inv_J2_omega1-h*Lern_inv_J1*j_inv_J2_omega1*Grad_Reib1-(h*Lern_inv_J1*Lern_c+Lern_inv_J1*Lern_d)*Grad_alpha_out_inv_J2;
j_c_omega1=(1+h*l1)*j_c_omega1-h*Lern_inv_J1*j_c_omega1*Grad_Reib1-h*Lern_inv_J1*delta_alpha_out-(h*Lern_inv_J1*Lern_c+Lern_inv_J1*Lern_d)*Grad_alpha_out_c;
j_d_omega1=(1+h*l1)*j_d_omega1-h*Lern_inv_J1*j_d_omega1*Grad_Reib1-Lern_inv_J1*delta_alpha_out-(h*Lern_inv_J1*Lern_c+Lern_inv_J1*Lern_d)*Grad_alpha_out_d;
j_Reib1_omega1=(1+h.*l1).*j_Reib1_omega1-h.*Lern_inv_J1.*(AF_GRNN(omega1,ksi)+j_Reib1_omega1.*Grad_Reib1)-(h.*Lern_inv_J1.*Lern_c+Lern_inv_J1.*Lern_d).*Grad_alpha_out_Reib1;
j_Reib2_omega1=(1+h.*l1).*j_Reib2_omega1-h.*Lern_inv_J1.*j_Reib2_omega1.*Grad_Reib1-(h.*Lern_inv_J1.*Lern_c+Lern_inv_J1.*Lern_d).*Grad_alpha_out_Reib2;
j_L_omega1=(1+h*l1)*j_L_omega1-h*Lern_inv_J1*j_L_omega1*Grad_Reib1-(h*Lern_inv_J1*Lern_c+Lern_inv_J1*Lern_d)*Grad_alpha_out_L;

end
